simulink model "CoherenceCalculation"  (R2016b)
settings: Solver=FixedStepAuto  StartTime=0.0  StopTime=inf  FixedStep=sCoreParams.core.stepPeriod*50  RelTol=1e-3  SampleTimeConstraint=STIndependent  EnableMultiTasking=on
undefined symbols (not defined in the file): sCoreParams, sCoreParams_decoders_txDetector_detectChannelInds
settings Model: Creator=anish  LastModifiedBy=rzelmann
settings SolverCC: EnableConcurrentExecution=on
settings DataIOCC: SaveFormat=StructureWithTime  SignalLoggingSaveFormat=ModelDataLogs  SaveOutput=off  SignalLogging=off  DSMLogging=off  SaveTime=off
settings OptimizationCC: BlockReduction=off  ConditionallyExecuteInputs=off  DefaultParameterBehavior=Inlined  OptimizeBlockIOStorage=off  BufferReuse=off  GlobalBufferReuse=off  ExpressionFolding=off  LocalBlockOutputs=off  LifeSpan=inf
settings DebuggingCC: SignalRangeChecking=error  SaveWithParameterizedLinksMsg=none  AllowSymbolicDim=off  ModelReferenceSymbolNameMessage=none  StateNameClashWarn=warning  SFUnexpectedBacktrackingDiag=warning  SFNoUnconditionalDefaultTransitionDiag=warning  SFExecutionAtInitializationDiag=none
settings HardwareCC: ProdBitPerPointer=32  ProdBitPerSizeT=32  ProdBitPerPtrDiffT=32  ProdLargestAtomicFloat=None  ProdWordSize=32  ProdLongLongMode=on  ProdHWDeviceType=Generic->32-bit x86 compatible  TargetBitPerPointer=64  TargetLargestAtomicFloat=Float  TargetLongLongMode=on  TargetIntDivRoundTo=Zero  TargetEndianess=LittleEndian  TargetWordSize=64  TargetHWDeviceType=Intel->x86-64 (Windows64)
settings ModelReferenceCC: UpdateModelReferenceTargets=Force  ModelReferenceNumInstancesAllowed=Single  ModelReferencePassRootInputsByReference=off
settings RTWCC: SystemTargetFile=slrt.tlc  TemplateMakefile=slrt_default_tmf  Description=Simulink Real-Time  BuildConfiguration=Faster Runs  RTWCompilerOptimization=on
settings TargetCC: CodeReplacementLibrary=XPC_BLAS  ParMdlRefBuildCompliant=on  ConcurrentExecutionCompliant=on  GeneratePreprocessorConditionals=Use local settings  MatFileLogging=on  MATLABClassNameForMDSCustomization=xpcAperiodicCustomization
settings ConfigComp: CovMetricSettings=dw  CovHtmlReporting=on  CovSaveCumulativeToWorkspaceVar=on  CovSaveSingleToWorkspaceVar=on  CovExternalEMLEnable=off  CovSFcnEnable=off

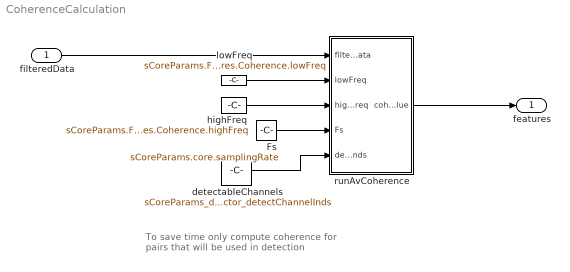
== system CoherenceCalculation ==
  note: To save time only compute coherence
      | for pairs that will be used in detection
  filteredData : Inport  PortDimensions=[sCoreParams.Features.Coherence.WindowDurationSamples sCoreParams.decoders.txDetector.nFilteredChannels]
  Fs : Constant  Value=sCoreParams.core.samplingRate
  detectableChannels : Constant  Value=sCoreParams_decoders_txDetector_detectChannelInds
  highFreq : Constant  Value=sCoreParams.Features.Coherence.highFreq
  lowFreq : Constant  Value=sCoreParams.Features.Coherence.lowFreq
  runAvCoherence : MATLAB Function  TreatAsAtomicUnit=on
  features : Outport
  wires:
  runAvCoherence/1(coherenceValue) -> features/1
  lowFreq/1 -> runAvCoherence/2(lowFreq)
  highFreq/1 -> runAvCoherence/3(highFreq)
  Fs/1 -> runAvCoherence/4(Fs)
  filteredData/1 -> runAvCoherence/1(filteredData)
  detectableChannels/1 -> runAvCoherence/5(detectChannelInds)

== matlab function CoherenceCalculation/runAvCoherence ==
  data: filteredData input; coherenceValue output; lowFreq input; highFreq input; Fs input; detectChannelInds input
function coherenceValue   = runCoherence(filteredData,  lowFreq, highFreq, Fs, detectChannelInds)
%#codegen
% Run mscohere in filteredData
% Returns magnitude-square coherence between pairs of channels for the whole time window
% coder.extrinsic('mscohere');
% freqBins = linspace(lowFreq, highFreq, 64);
% [coherenceValue1, fValues] = mscohere(filteredData, filteredData, [], [], freqBins, Fs);
% avCoherence1 = mean(coherenceValue1(:));    % average across all intereactions

%[~, avCoherence, coherenceValue, pairChannels] = runCoherence_EML(filteredData, lowFreq, highFreq, Fs, detectChannelInds);
[~, avCoherence, coherenceValue, pairChannels] = runCoherence_NoDownsampling_EML(filteredData, lowFreq, highFreq, Fs, detectChannelInds);
%[sumCoherencePerChannel, avCoherence, coherenceValue] = runCoherenceMultitaper_EML(filteredData, lowFreq, highFreq, nPoints, Fs);
